simulink model "LQR_linear_model"  (R2022a)
settings: Solver=VariableStepAuto  StartTime=0.0  StopTime=Tmax  RelTol=1e-3
values from neighbouring files (symbols this model uses):
  Ad = sysd.A    [Ex4.m]    (also in Ex5.m; systeem.mat = [1 0 0 0 0 0 0 0 0 0 0 0 ... (144 elements, 12x12)])
  Bd = sysd.B    [Ex4.m]    (also in Ex5.m; systeem.mat = [0 -5.07773769891e-05 0.00033126933 0 -0.00203109507956 0.01)
  Cd = sysd.C    [Ex4.m]    (also in Ex5.m; systeem.mat = [0.22360679775 0 0 0 0 0 0 0 0 0 0 0 ... (144 elements, 12x1)
  Dd = sysd.D    [Ex4.m]    (also in Ex5.m; systeem.mat = [0 -5.67708333333e-06 3.7037037037e-05 0 -0.000227083333333 )
  K = dlqr(Ad,Bd,Q,R)    [Ex3.m]    (also in rscale.m = k)
  Nu = N(13:end,:)    [Ex5.m]    (also in rscale.m = N(s1:end,:))
  Nx = N(1:12,:)    [Ex5.m]    (also in rscale.m = N(1:s1(1),:))
  Ts = 0.05    [Ex2.m]    (also in Ex3.m; Ex4.m; Ex5.m)
settings Model: Creator=ninac  LastModifiedBy=Nina Claessens
settings DebuggingCC: UnconnectedInputMsg=warning  UnconnectedOutputMsg=warning  UnconnectedLineMsg=warning
settings RTWCC: DLArmComputeVersion=19.05

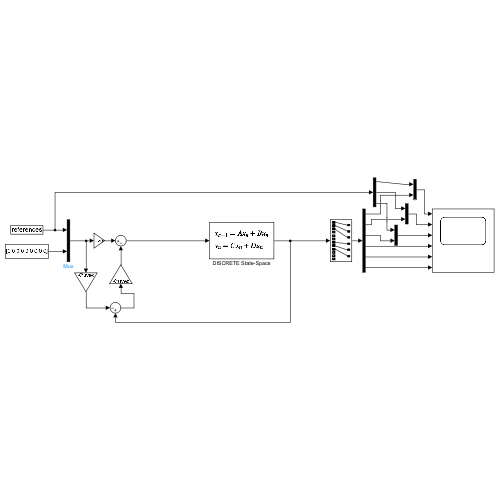
[thumbnail: Simulink's stored preview of the top-level diagram]
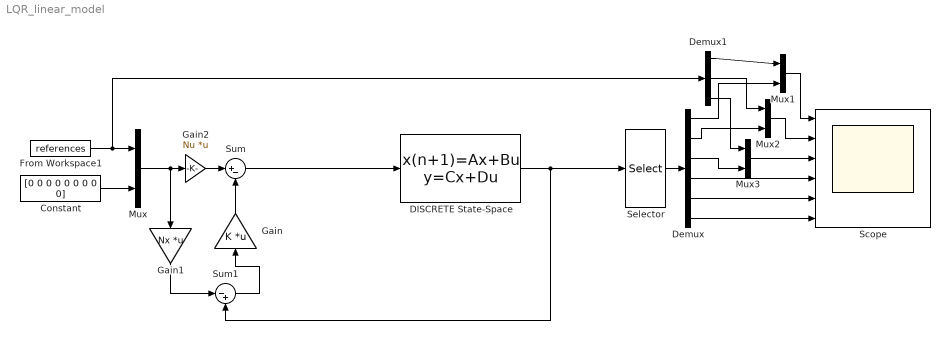
== system LQR_linear_model ==
  Constant : Constant  Value=[0 0 0 0 0 0 0 0 0]  SampleTime=Ts
  DISCRETE State-Space : DiscreteStateSpace  A=Ad  B=Bd  C=Cd  D=Dd  SampleTime=Ts
  Demux : Demux  Outputs=6
  Demux1 : Demux  Outputs=3
  From Workspace1 : FromWorkspace  VariableName=references  SampleTime=Ts  Interpolate=off  OutputAfterFinalValue=Holding final value
  Gain : Gain  Gain=K  Multiplication=Matrix(K*u) (u vector)
  Gain1 : Gain  Gain=Nx  Multiplication=Matrix(K*u) (u vector)
  Gain2 : Gain  Gain=Nu  Multiplication=Matrix(K*u) (u vector)
  Mux{,1..3} (4 alike) : Mux  Inputs=2
  Scope : Scope  NumInputPorts=6
  Selector : Selector  InputPortWidth=12  IndexOptions=Index vector (dialog)  Indices=[1 2 3 7 8 9]  OutputSizes=1
  Sum : Sum  Inputs=|+-
  Sum1 : Sum  Inputs=|-+
  wires:
  Mux/1 -> Gain1/1, Gain2/1
  DISCRETE State-Space/1 -> Sum1/2, Selector/1
  From Workspace1/1 -> Demux1/1, Mux/1
  Constant/1 -> Mux/2
  Selector/1 -> Demux/1
  Demux/1 -> Mux1/2
  Demux/2 -> Mux2/2
  Demux/3 -> Mux3/2
  Demux/4 -> Scope/4
  Demux/5 -> Scope/5
  Demux/6 -> Scope/6
  Demux1/1 -> Mux1/1
  Mux1/1 -> Scope/1
  Demux1/2 -> Mux2/1
  Mux2/1 -> Scope/2
  Demux1/3 -> Mux3/1
  Mux3/1 -> Scope/3
  Gain/1 -> Sum/2
  Sum/1 -> DISCRETE State-Space/1
  Sum1/1 -> Gain/1
  Gain1/1 -> Sum1/1
  Gain2/1 -> Sum/1
